simulink model "RRRplanaire"  (R2023a)
settings: Solver=ode23  StartTime=0.0  StopTime=10  FixedStep=.1  RelTol=1e-3  EnableMultiTasking=on
values from neighbouring files (symbols this model uses):
  A = 0.1    [Boucle.m]    (also in param.m)
  w = 1    [Boucle.m]    (also in param.m)
  x0 = 0.4    [Boucle.m]    (also in param.m)
  y0 = 0.3    [Boucle.m]    (also in param.m)
libraries: vrlib x4, dspsolvers x1
settings Model: Creator=dgarcia  LastModifiedBy=maxim
settings SolverCC: AlgebraicLoopSolver=TrustRegion
settings DataIOCC: LimitDataPoints=on  SaveFormat=Array  SignalLoggingSaveFormat=ModelDataLogs  ReturnWorkspaceOutputs=off  SignalLoggingName=sigsOut
settings OptimizationCC: ExpressionDepthLimit=2147483647  InitFltsAndDblsToZero=on  LifeSpan=inf
settings DebuggingCC: SaveWithParameterizedLinksMsg=none  UnderspecifiedInitializationDetection=Classic  MergeDetectMultiDrivingBlocksExec=none  SignalResolutionControl=TryResolveAllWithWarning  MultiTaskDSMMsg=warning  MultiTaskCondExecSysMsg=none  FcnCallInpInsideContextMsg=warning  UnconnectedInputMsg=warning  UnconnectedOutputMsg=warning  UnconnectedLineMsg=warning  StateNameClashWarn=warning  SFUnexpectedBacktrackingDiag=warning  SFNoUnconditionalDefaultTransitionDiag=warning  ArithmeticOperatorsInVariantConditions=warning
settings HardwareCC: ProdBitPerPointer=32  ProdBitPerSizeT=32  ProdBitPerPtrDiffT=32  ProdLargestAtomicFloat=None  ProdIntDivRoundTo=Undefined  ProdEndianess=Unspecified  ProdWordSize=32  ProdHWDeviceType=32-bit Generic  TargetUnknown=on
settings ModelReferenceCC: EnableRefExpFcnMdlSchedulingChecks=on  PropagateSignalLabelsOutOfModel=off
settings SFSimCC: SimUseLocalCustomCode=off  SimParseCustomCode=off  CustomCodeUndefinedFunction=UseInterfaceOnly
settings RTWCC: RTWUseLocalCustomCode=off  DLArmComputeVersion=19.05
settings CodeAppCC: StateflowObjectComments=on
settings GRTTargetCC: TargetFcnLib=ansi_tfl_tmw.mat  TargetLangStandard=C89/C90 (ANSI)  CombineOutputUpdateFcns=off  GRTInterface=on
settings ConfigComp: CovMetricSettings=dw  CovSaveCumulativeToWorkspaceVar=on  CovSaveSingleToWorkspaceVar=on  CovExternalEMLEnable=off

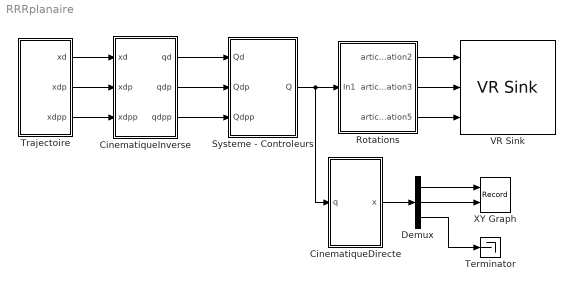
== system RRRplanaire ==
  CinematiqueDirecte : Subsystem
  CinematiqueInverse : Subsystem
  Demux : Demux  Outputs=3
  Rotations : Subsystem
  Systeme - Controleurs : Subsystem
  Terminator : Terminator
  Trajectoire : Subsystem
  VR Sink : vrlib/VR Sink  InstantiateOnLoad=on  SampleTime=0.1  ViewEnable=on  RemoteChange=off  RemoteView=on  FieldsWritten=Joint2.rotation.4.1.double#Joint3.rotation.4.1.double#Joint5.rotation.4.1.double  WorldFileName=LRMate200iC.wrl  AutoView=off  VideoDimensions=[]  AllowVariableSize=off
  XY Graph : Record  FileSettingsInternal="{\"entries\":[{\"content\":{\"excelSettings\":{\"content\":{},\"type\":\"Streamout.ExcelSettings\"}},\"type\":\"Streamout.FileSettingStorage\",\"uuid\":\"15e78eb5-29a8-49a9-9840-80e2d80b59b9\"}],\"packageUris\":[\"http://schema.mathworks.com/mf0/streamout_blocks/R2020a\"],\"version\":\"1.0\"}"  Layout=[1 1]  SignalsInternal="{\"entries\":[{\"content\":{\"signals\":[{\"content\":{\"blockPath\":[\"RRRplanaire/XY Graph\"],\"dimensions\":[1],\"domain\":\"RRRplanaire/XY Graph\",\"lineColor\":\"#a2142f\",\"plots\":[1],\"port\":1,\"signalID\":16,\"signalName\":\"XY Graph:1\"},\"type\":\"RecordBlkView.Signal\",\"uuid\":\"495b3c76-def4-49bc-ad31-84cb6030c742\"},{\"content\":{\"blockPath\":[\"RRRplanaire/XY Graph\"],\"dimensions\":[1],\"domain\":\"RRRplanaire/XY Graph\",\"lineColor\":\"#139fff\",\"plots\":[1],\"port\":2,\"signalID\":19,\"signalName\":\"XY Graph:2\"},\"type\":\"RecordBlkView.Signal\",\"uuid\":\"4d725a8f-b7c2-4f23-bdfe-d8f8ae9227f4\"}]},\"type\":\"RecordBlkView.InputSignals\",\"uuid\":\"0fe62230-b389-4f09-ad52-d3f22d0d1e4d\"}],\"packageUris\":[\"http://schema.mathworks.com/mf0/streamout_blocks/R2020a\"],\"version\":\"1.0\"}"  VisualizationBindings="{\"xyplotplugin\":{\"info\":[{\"series\":[{\"bindingParametersList\":[{\"parameter\":\"X-Axis\",\"signalID\":16,\"signalName\":\"XY Graph:1\"},{\"parameter\":\"Y-Axis\",\"signalID\":19,\"signalName\":\"XY Graph:2\"}],\"seriesID\":11629}],\"subplotID\":1}]}}"  CompatibilityTag=XY  st=-1
  wires:
  Systeme - Controleurs/1(Q) -> CinematiqueDirecte/1(q), Rotations/1(In1)
  Trajectoire/1(xd) -> CinematiqueInverse/1(xd)
  Trajectoire/3(xdpp) -> CinematiqueInverse/3(xdpp)
  CinematiqueInverse/3(qdpp) -> Systeme - Controleurs/3(Qdpp)
  Trajectoire/2(xdp) -> CinematiqueInverse/2(xdp)
  CinematiqueInverse/1(qd) -> Systeme - Controleurs/1(Qd)
  CinematiqueInverse/2(qdp) -> Systeme - Controleurs/2(Qdp)
  CinematiqueDirecte/1(x) -> Demux/1
  Demux/1 -> XY Graph/1
  Demux/2 -> XY Graph/2
  Demux/3 -> Terminator/1
  Rotations/1(articulation2) -> VR Sink/1
  Rotations/2(articulation3) -> VR Sink/2
  Rotations/3(articulation5) -> VR Sink/3

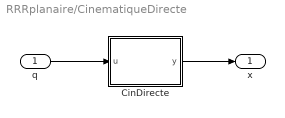
== system RRRplanaire/CinematiqueDirecte ==
  q : Inport
  CinDirecte : MATLAB Function  TreatAsAtomicUnit=on
  x : Outport
  wires:
  q/1 -> CinDirecte/1(u)
  CinDirecte/1(y) -> x/1

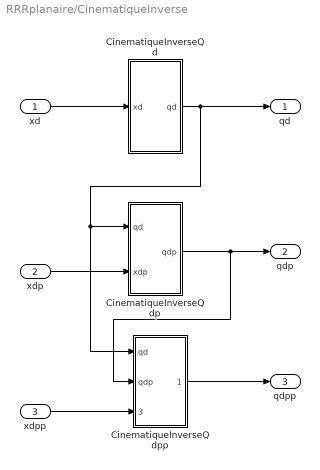
== system RRRplanaire/CinematiqueInverse ==
  xd : Inport
  xdp : Inport  Port=2
  xdpp : Inport  Port=3
  CinematiqueInverseQd : Subsystem
  CinematiqueInverseQdp : Subsystem
  CinematiqueInverseQdpp : Subsystem
  qd : Outport
  qdp : Outport  Port=2
  qdpp : Outport  Port=3
  wires:
  CinematiqueInverseQd/1(qd) -> CinematiqueInverseQdp/1(qd), CinematiqueInverseQdpp/1(qd), qd/1
  xdp/1 -> CinematiqueInverseQdp/2(xdp)
  CinematiqueInverseQdp/1(qdp) -> qdp/1, CinematiqueInverseQdpp/2(qdp)
  xd/1 -> CinematiqueInverseQd/1(xd)
  CinematiqueInverseQdpp/1(qdpp) -> qdpp/1
  xdpp/1 -> CinematiqueInverseQdpp/3(xdpp)

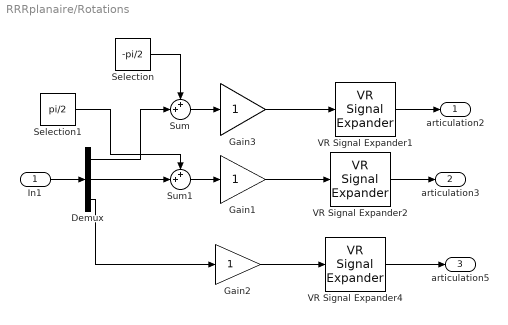
== system RRRplanaire/Rotations ==
  In1 : Inport
  Demux : Demux  Outputs=3
      settings: DisplayOption=none
  Gain1 : Gain
  Gain2 : Gain
  Gain3 : Gain
  Selection : Constant  Value=-pi/2  VectorParams1D=off
  Selection1 : Constant  Value=pi/2  VectorParams1D=off
  Sum : Sum  Inputs=++|
  Sum1 : Sum  Inputs=++|
  VR Signal Expander1 : vrlib/VR Signal Expander  outwidth=4  outidx=4
  VR Signal Expander2 : vrlib/VR Signal Expander  outwidth=4  outidx=4
  VR Signal Expander4 : vrlib/VR Signal Expander  outwidth=4  outidx=4
  articulation2 : Outport
  articulation3 : Outport  Port=2
  articulation5 : Outport  Port=3
  wires:
  In1/1 -> Demux/1
  VR Signal Expander1/1 -> articulation2/1
  VR Signal Expander2/1 -> articulation3/1
  Gain1/1 -> VR Signal Expander2/1
  Gain3/1 -> VR Signal Expander1/1
  VR Signal Expander4/1 -> articulation5/1
  Demux/3 -> Gain2/1
  Gain2/1 -> VR Signal Expander4/1
  Selection/1 -> Sum/1
  Demux/1 -> Sum/2
  Sum/1 -> Gain3/1
  Demux/2 -> Sum1/2
  Sum1/1 -> Gain1/1
  Selection1/1 -> Sum1/1

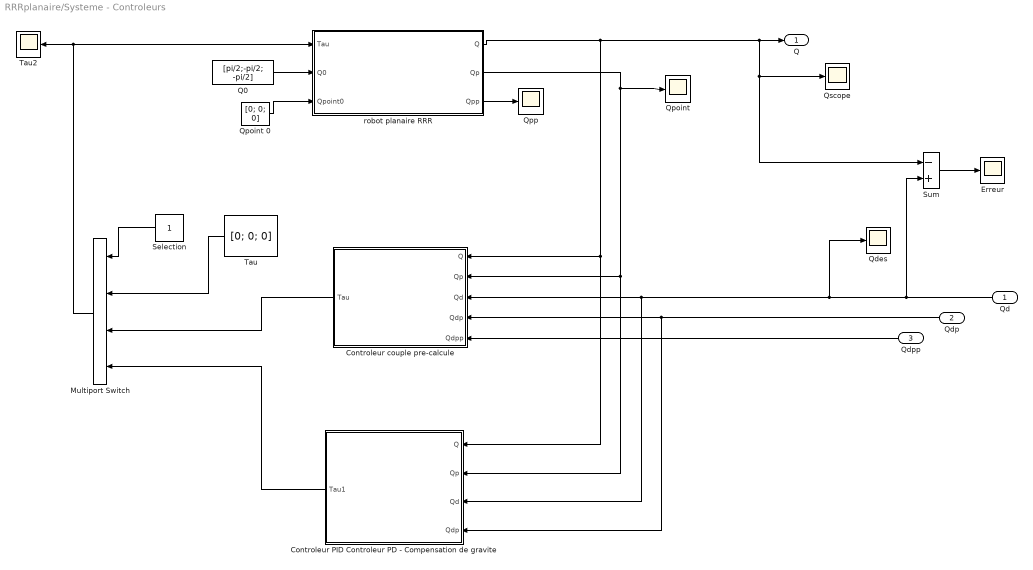
== system RRRplanaire/Systeme - Controleurs ==
  Qd : Inport
  Qdp : Inport  Port=2
  Qdpp : Inport  Port=3
  Controleur PID Controleur PD - Compensation de gravite : Subsystem
  Controleur couple pre-calcule : Subsystem
  Erreur : Scope
  Multiport Switch : MultiPortSwitch  InputSameDT=off
  "Q0 " : Constant  Value=[pi/2;-pi/2; -pi/2]  VectorParams1D=off
  Qdes : Scope
  Qpoint : Scope
  "Qpoint 0  " : Constant  Value=[0; 0; 0]  VectorParams1D=off
  Qpp : Scope
  Qscope : Scope
  Selection : Constant  VectorParams1D=off
  Sum : Sum  Inputs=-+  SaturateOnIntegerOverflow=on
  Tau : Constant  Value=[0; 0; 0]  VectorParams1D=off
  Tau2 : Scope
  robot planaire RRR : Subsystem
  Q : Outport
  wires:
  "Q0 "/1 -> robot planaire RRR/2(Q0)
  "Qpoint 0  "/1 -> robot planaire RRR/3(Qpoint0)
  robot planaire RRR/1(Q) -> Sum/1, Qscope/1, Q/1, Controleur couple pre-calcule/1(Q), Controleur PID Controleur PD - Compensation de gravite/1(Q)
  robot planaire RRR/2(Qp) -> Qpoint/1, Controleur PID Controleur PD - Compensation de gravite/2(Qp), Controleur couple pre-calcule/2(Qp)
  Sum/1 -> Erreur/1
  Controleur couple pre-calcule/1(Tau) -> Multiport Switch/3
  Tau/1 -> Multiport Switch/2
  Selection/1 -> Multiport Switch/1
  Controleur PID Controleur PD - Compensation de gravite/1(Tau1) -> Multiport Switch/4
  Qd/1 -> Sum/2, Controleur couple pre-calcule/3(Qd), Controleur PID Controleur PD - Compensation de gravite/3(Qd), Qdes/1
  Multiport Switch/1 -> Tau2/1, robot planaire RRR/1(Tau)
  Qdp/1 -> Controleur couple pre-calcule/4(Qdp), Controleur PID Controleur PD - Compensation de gravite/4(Qdp)
  Qdpp/1 -> Controleur couple pre-calcule/5(Qdpp)
  robot planaire RRR/3(Qpp) -> Qpp/1

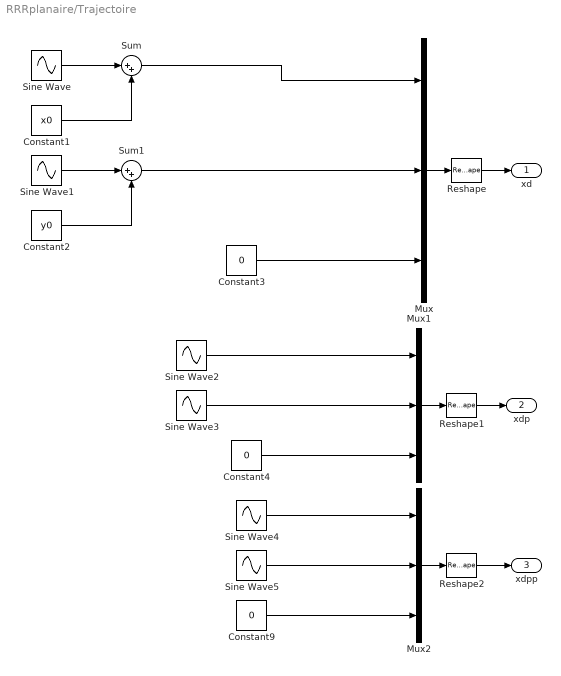
== system RRRplanaire/Trajectoire ==
  Constant1 : Constant  Value=x0
  Constant2 : Constant  Value=y0
  Constant3 : Constant  Value=0
  Constant4 : Constant  Value=0
  Constant9 : Constant  Value=0
  Mux : Mux  Inputs=3
  Mux1 : Mux  Inputs=3
  Mux2 : Mux  Inputs=3
  Reshape : Reshape  OutputDimensionality=Column vector (2-D)
  Reshape1 : Reshape  OutputDimensionality=Column vector (2-D)
  Reshape2 : Reshape  OutputDimensionality=Column vector (2-D)
  Sine Wave : Sin  Amplitude=A  Frequency=w  Phase=-pi/2  SampleTime=0
  Sine Wave1 : Sin  Amplitude=A  Frequency=w  SampleTime=0
  Sine Wave2 : Sin  Amplitude=-A*w  Frequency=w  SampleTime=0
  Sine Wave3 : Sin  Amplitude=A*w  Frequency=w  Phase=-pi/2  SampleTime=0
  Sine Wave4 : Sin  Amplitude=-A*w^2  Frequency=w  Phase=-pi/2  SampleTime=0
  Sine Wave5 : Sin  Amplitude=-A*w^2  Frequency=w  SampleTime=0
  Sum : Sum  Inputs=|++
  Sum1 : Sum  Inputs=|++
  xd : Outport
  xdp : Outport  Port=2
  xdpp : Outport  Port=3
  wires:
  Mux/1 -> Reshape/1
  Mux1/1 -> Reshape1/1
  Mux2/1 -> Reshape2/1
  Reshape/1 -> xd/1
  Reshape1/1 -> xdp/1
  Reshape2/1 -> xdpp/1
  Sum1/1 -> Mux/2
  Constant3/1 -> Mux/3
  Sine Wave2/1 -> Mux1/1
  Sine Wave3/1 -> Mux1/2
  Sine Wave4/1 -> Mux2/1
  Sine Wave5/1 -> Mux2/2
  Constant9/1 -> Mux2/3
  Constant1/1 -> Sum/2
  Sine Wave/1 -> Sum/1
  Sum/1 -> Mux/1
  Sine Wave1/1 -> Sum1/1
  Constant2/1 -> Sum1/2
  Constant4/1 -> Mux1/3

== system RRRplanaire/CinematiqueInverse/CinematiqueInverseQd ==
  xd : Inport
  q2 : MATLAB Function  TreatAsAtomicUnit=on
  qd : Outport
  wires:
  q2/1(y) -> qd/1
  xd/1 -> q2/1(u)

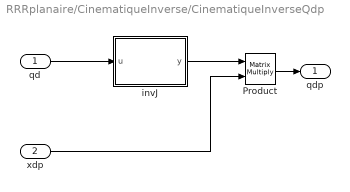
== system RRRplanaire/CinematiqueInverse/CinematiqueInverseQdp ==
  qd : Inport
  xdp : Inport  Port=2
  Product : Product  Multiplication=Matrix(*)  RndMeth=Zero
  invJ : MATLAB Function  TreatAsAtomicUnit=on
  qdp : Outport
  wires:
  xdp/1 -> Product/2
  qd/1 -> invJ/1(u)
  invJ/1(y) -> Product/1
  Product/1 -> qdp/1

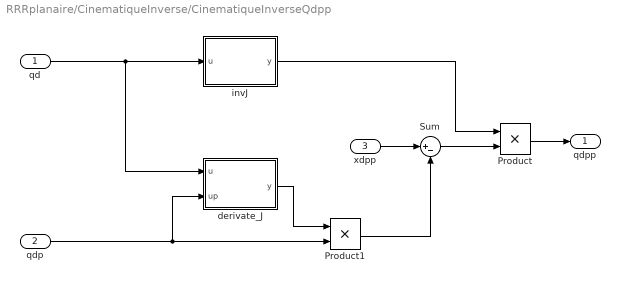
== system RRRplanaire/CinematiqueInverse/CinematiqueInverseQdpp ==
  qd : Inport
  qdp : Inport  Port=2
  xdpp : Inport  Port=3
  Product : Product
  Product1 : Product
  Sum : Sum  Inputs=|+-
  derivate_J : MATLAB Function  TreatAsAtomicUnit=on
  invJ : MATLAB Function  TreatAsAtomicUnit=on
  qdpp : Outport
  wires:
  qd/1 -> invJ/1(u), derivate_J/1(u)
  qdp/1 -> Product1/2, derivate_J/2(up)
  Product/1 -> qdpp/1
  xdpp/1 -> Sum/1
  derivate_J/1(y) -> Product1/1
  Product1/1 -> Sum/2
  Sum/1 -> Product/2
  invJ/1(y) -> Product/1

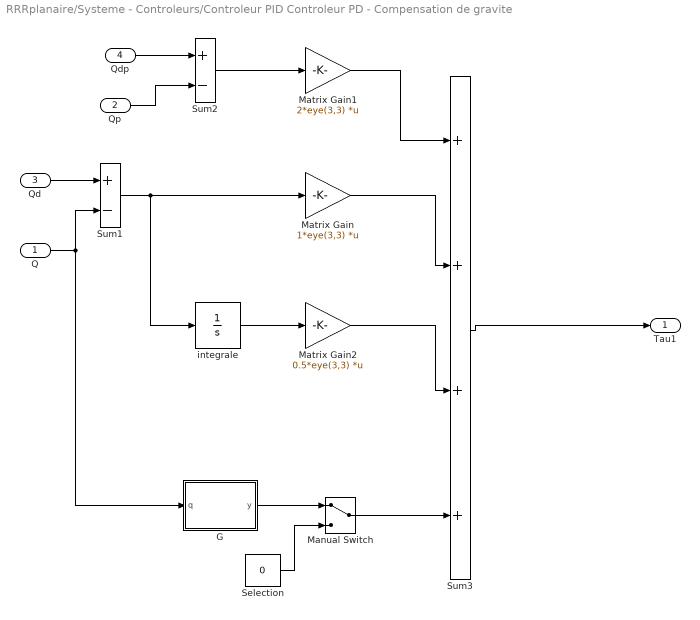
== system RRRplanaire/Systeme - Controleurs/Controleur PID Controleur PD - Compensation de gravite ==
  Q : Inport
  Qp : Inport  Port=2
  Qd : Inport  Port=3
  Qdp : Inport  Port=4
  G : MATLAB Function  TreatAsAtomicUnit=on
  Manual Switch : ManualSwitch
  Matrix Gain : Gain  Gain=1*eye(3,3)  Multiplication=Matrix(K*u)  SaturateOnIntegerOverflow=on  OutDataTypeStr=Inherit: Same as input  ParamDataTypeStr=Inherit: Same as input
  Matrix Gain1 : Gain  Gain=2*eye(3,3)  Multiplication=Matrix(K*u)  SaturateOnIntegerOverflow=on  OutDataTypeStr=Inherit: Same as input  ParamDataTypeStr=Inherit: Same as input
  Matrix Gain2 : Gain  Gain=0.5*eye(3,3)  Multiplication=Matrix(K*u)  SaturateOnIntegerOverflow=on  OutDataTypeStr=Inherit: Same as input  ParamDataTypeStr=Inherit: Same as input
  Selection : Constant  Value=0  VectorParams1D=off
  Sum1 : Sum  Inputs=+-  InputSameDT=on  SaturateOnIntegerOverflow=on  OutDataTypeStr=Inherit: Same as first input
  Sum2 : Sum  Inputs=+-  InputSameDT=on  SaturateOnIntegerOverflow=on  OutDataTypeStr=Inherit: Same as first input
  Sum3 : Sum  Inputs=++++  InputSameDT=on  SaturateOnIntegerOverflow=on  OutDataTypeStr=Inherit: Same as first input
  integrale : Integrator  InitialCondition=[0; 0; 0]
  Tau1 : Outport
  wires:
  Selection/1 -> Manual Switch/2
  G/1(y) -> Manual Switch/1
  Manual Switch/1 -> Sum3/4
  Sum3/1 -> Tau1/1
  Matrix Gain2/1 -> Sum3/3
  Matrix Gain/1 -> Sum3/2
  Matrix Gain1/1 -> Sum3/1
  integrale/1 -> Matrix Gain2/1
  Qdp/1 -> Sum2/1
  Sum2/1 -> Matrix Gain1/1
  Sum1/1 -> integrale/1, Matrix Gain/1
  Qd/1 -> Sum1/1
  Qp/1 -> Sum2/2
  Q/1 -> G/1(q), Sum1/2

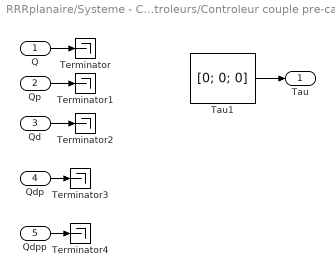
== system RRRplanaire/Systeme - Controleurs/Controleur couple pre-calcule ==
  Q : Inport
  Qp : Inport  Port=2
  Qd : Inport  Port=3
  Qdp : Inport  Port=4
  Qdpp : Inport  Port=5
  Tau1 : Constant  Value=[0; 0; 0]  VectorParams1D=off
  Terminator{,1..4} (5 alike) : Terminator
  Tau : Outport
  wires:
  Qdpp/1 -> Terminator4/1
  Qdp/1 -> Terminator3/1
  Q/1 -> Terminator/1
  Qp/1 -> Terminator1/1
  Qd/1 -> Terminator2/1
  Tau1/1 -> Tau/1

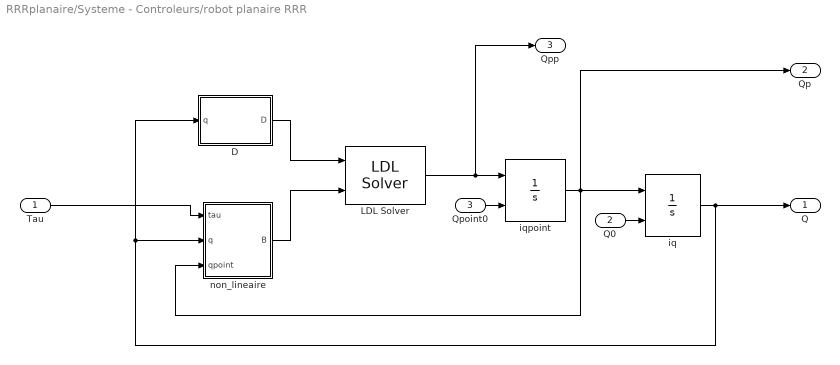
== system RRRplanaire/Systeme - Controleurs/robot planaire RRR ==
  Tau : Inport
  Q0 : Inport  Port=2
  Qpoint0 : Inport  Port=3
  "D " : MATLAB Function  TreatAsAtomicUnit=on
  LDL Solver : dspsolvers/LDL Solver  errmode=Warning
  iq : Integrator  InitialConditionSource=external  InitialCondition=[0;-pi/2; 0]
  iqpoint : Integrator  InitialConditionSource=external  InitialCondition=[0; 0; 0]
  non_lineaire : Subsystem
  Q : Outport
  Qp : Outport  Port=2
  Qpp : Outport  Port=3
  wires:
  "D "/1(D) -> LDL Solver/1
  non_lineaire/1(B) -> LDL Solver/2
  LDL Solver/1 -> iqpoint/1, Qpp/1
  iq/1 -> "D "/1(q), non_lineaire/2(q), Q/1
  Q0/1 -> iq/2
  iqpoint/1 -> iq/1, Qp/1, non_lineaire/3(qpoint)
  Qpoint0/1 -> iqpoint/2
  Tau/1 -> non_lineaire/1("tau ")

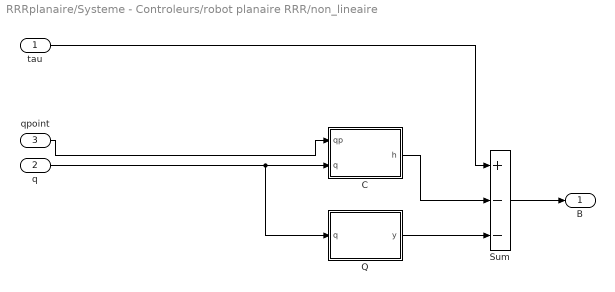
== system RRRplanaire/Systeme - Controleurs/robot planaire RRR/non_lineaire ==
  "tau " : Inport
  q : Inport  Port=2
  qpoint : Inport  Port=3
  C : MATLAB Function  TreatAsAtomicUnit=on
  "Q " : MATLAB Function  TreatAsAtomicUnit=on
  Sum : Sum  Inputs=+--  InputSameDT=on  SaturateOnIntegerOverflow=on  OutDataTypeStr=Inherit: Same as first input
  B : Outport
  wires:
  q/1 -> "Q "/1(q), C/2(q)
  "tau "/1 -> Sum/1
  Sum/1 -> B/1
  "Q "/1(y) -> Sum/3
  C/1(h) -> Sum/2
  qpoint/1 -> C/1(qp)

== matlab function RRRplanaire/Systeme - Controleurs/Controleur PID Controleur PD - Compensation de gravite/G ==
  data: q input; y output
function y = fcn(q)

% Paramètres
M1 = 1;
M2 = 1;
M3 = 0.5;
L1 = 300*0.001;
L2 = 320*0.001;
L3 = 80*0.001;
g = 9.81;
T = 0.01;


I1 = 1/12*M1*L1^2;
I2 = 1/12*M2*L2^2;
I3 = 1/12*M3*L3^2;
C1 = L1/2;
C2 = L2/2;
C3 = L3/2;
p1 = M1*C1^2+I1+(M2+M3)*L1^2;
p2 = M2*C2^2+I2+M3*L2^2;
p3 = M3*C3^2+I3;
p4 = (M2+2*M3)*L1*L2/2;
p5 = M3*L1*L3/2;
p6 = M3*L2*L3/2;
p7 = (M1*C1+(M2+M3)*L1)*g;
p8 = (M2*C2+M3*L2)*g;
p9 = M3*C3*g;

y = [p7*cos(q(1))+p8*cos(q(1)+q(2))+p9*cos(q(1)+q(2)+q(3))
     p8*cos(q(1)+q(2))+p9*cos(q(1)+q(2)+q(3))
     p9*cos(q(1)+q(2)+q(3))];

== matlab function RRRplanaire/CinematiqueInverse/CinematiqueInverseQdpp/derivate_J ==
  data: u input; y output; up input
function y = fcn(u,up)

% Paramètres
L1 = 300*0.001;
L2 = 320*0.001;
L3 = 80*0.001;

y=[-L3 * cos(u(1) + u(2) + u(3))*(up(1)+up(2)+up(3)) - L2 * cos(u(1) + u(2))*(up(1)+up(2)) - L1 * cos(u(1))*up(1), -L3 * cos(u(1) + u(2) + u(3))*(up(1)+up(2)+up(3)) - L2 * cos(u(1) + u(2))*(up(1)+up(2)), -L3 * cos(u(1) + u(2) + u(3))*(up(1)+up(2)+up(3)); 
   -L3 * sin(u(1) + u(2) + u(3))*(up(1)+up(2)+up(3)) - L2 * sin(u(1) + u(2))*(up(1)+up(2)) - L1 * sin(u(1))*up(1), -L3 * sin(u(1) + u(2) + u(3))*(up(1)+up(2)+up(3)) - L2 * sin(u(1) + u(2))*(up(1)+up(2)), -L3 * sin(u(1) + u(2) + u(3))*(up(1)+up(2)+up(3));
   1 1 1;];

== matlab function RRRplanaire/Systeme - Controleurs/robot planaire RRR/D  ==
  data: q input; D output
function D = fcn(q)

% Paramètres
M1 = 1;
M2 = 1;
M3 = 0.5;
L1 = 300*0.001;
L2 = 320*0.001;
L3 = 80*0.001;
g = 9.81;
T = 0.01;

I1 = 1/12*M1*L1^2;
I2 = 1/12*M2*L2^2;
I3 = 1/12*M3*L3^2;
C1 = L1/2;
C2 = L2/2;
C3 = L3/2;
p1 = M1*C1^2+I1+(M2+M3)*L1^2;
p2 = M2*C2^2+I2+M3*L2^2;
p3 = M3*C3^2+I3;
p4 = (M2+2*M3)*L1*L2/2;
p5 = M3*L1*L3/2;
p6 = M3*L2*L3/2;
p7 = (M1*C1+(M2+M3)*L1)*g;
p8 = (M2*C2+M3*L2)*g;
p9 = M3*C3*g;

D = [p1+p2+p3+2*p4*cos(q(2))+2*p5*cos(q(2)+q(3))+2*p6*cos(q(3)) p2+p3+p4*cos(q(2))+p5*cos(q(2)+q(3))+2*p6*cos(q(3)) p3+p5*cos(q(2)+q(3))+p6*cos(q(3))
     p2+p3+p4*cos(q(2))+p5*cos(q(2)+q(3))+2*p6*cos(q(3)) p2+p3+2*p6*cos(q(3)) p3+p6*cos(q(3))
     p3+p5*cos(q(2)+q(3))+p6*cos(q(3)) p3+p6*cos(q(3)) p3];

== matlab function RRRplanaire/Systeme - Controleurs/robot planaire RRR/non_lineaire/C ==
  data: qp input; h output; q input
function h = fcn(qp,q)

% Paramètres
M1 = 1;
M2 = 1;
M3 = 0.5;
L1 = 300*0.001;
L2 = 320*0.001;
L3 = 80*0.001;
g = 9.81;
T = 0.01;

I1 = 1/12*M1*L1^2;
I2 = 1/12*M2*L2^2;
I3 = 1/12*M3*L3^2;
C1 = L1/2;
C2 = L2/2;
C3 = L3/2;
p1 = M1*C1^2+I1+(M2+M3)*L1^2;
p2 = M2*C2^2+I2+M3*L2^2;
p3 = M3*C3^2+I3;
p4 = (M2+2*M3)*L1*L2/2;
p5 = M3*L1*L3/2;
p6 = M3*L2*L3/2;
p7 = (M1*C1+(M2+M3)*L1)*g;
p8 = (M2*C2+M3*L2)*g;
p9 = M3*C3*g;

h = [-p4*(2*qp(1)+qp(2))*qp(2)*sin(q(2))-p5*(qp(2)+qp(3))*(2*qp(1)+qp(2)+qp(3))*sin(q(2)+q(3))-p6*qp(3)*(2*qp(1)+2*qp(2)+qp(3))*sin(q(3))
     p4*sin(q(2))*qp(1)^2+p5*sin(q(2)+q(3))*qp(1)^2-p6*(2*qp(1)+2*qp(2)+qp(3))*qp(3)*sin(q(3))
     p5*sin(q(2)+q(3))*qp(1)^2+p6*sin(q(3))*(qp(1)+qp(2))^2];

== matlab function RRRplanaire/Systeme - Controleurs/robot planaire RRR/non_lineaire/Q  ==
  data: q input; y output
function y = fcn(q)

% Paramètres
M1 = 1;
M2 = 1;
M3 = 0.5;
L1 = 300*0.001;
L2 = 320*0.001;
L3 = 80*0.001;
g = 9.81;
T = 0.01;

I1 = 1/12*M1*L1^2;
I2 = 1/12*M2*L2^2;
I3 = 1/12*M3*L3^2;
C1 = L1/2;
C2 = L2/2;
C3 = L3/2;
p1 = M1*C1^2+I1+(M2+M3)*L1^2;
p2 = M2*C2^2+I2+M3*L2^2;
p3 = M3*C3^2+I3;
p4 = (M2+2*M3)*L1*L2/2;
p5 = M3*L1*L3/2;
p6 = M3*L2*L3/2;
p7 = (M1*C1+(M2+M3)*L1)*g;
p8 = (M2*C2+M3*L2)*g;
p9 = M3*C3*g;

y = [p7*cos(q(1))+p8*cos(q(1)+q(2))+p9*cos(q(1)+q(2)+q(3))
     p8*cos(q(1)+q(2))+p9*cos(q(1)+q(2)+q(3))
     p9*cos(q(1)+q(2)+q(3))];

== matlab function RRRplanaire/CinematiqueInverse/CinematiqueInverseQd/q2 ==
  data: u input; y output
function y = fcn(u)
% u(1) = Ex_d, u(2) = Ey_d, u(3) = theta_d
% y(1) = theta(1), y(2) = theta(2), y(3) = theta(3)

% Paramètres
l1 = 300*0.001;
l2 = 320*0.001;
l3 = 80*0.001;

xd = u(1);
yd = u(2);
phi_des = u(3);
Wx = xd - l3*cos(phi_des);
Wy = yd - l3*sin(phi_des);
d = sqrt(Wx^2+Wy^2);
theta1 = atan2(Wy,Wx) + acos((d^2+l1^2-l2^2)/(2*d*l1));
theta2 = -acos((d^2-l1^2-l2^2)/(2*l1*l2));
theta3 = phi_des - theta2- theta1;

y=[theta1, theta2, theta3];

== matlab function RRRplanaire/CinematiqueInverse/CinematiqueInverseQdp/invJ ==
  data: u input; y output
function y = fcn(u)

% Paramètres
L1 = 300*0.001;
L2 = 320*0.001;
L3 = 80*0.001;

J=[-L3 * sin(u(1) + u(2) + u(3)) - L2 * sin(u(1) + u(2)) - L1 * sin(u(1)) -L3 * sin(u(1) + u(2) + u(3)) - L2 * sin(u(1) + u(2)) -L3 * sin(u(1) + u(2) + u(3)); L3 * cos(u(1) + u(2) + u(3)) + L2 * cos(u(1) + u(2)) + L1 * cos(u(1)) L3 * cos(u(1) + u(2) + u(3)) + L2 * cos(u(1) + u(2)) L3 * cos(u(1) + u(2) + u(3)); 1 1 1;];
y=inv(J);

== matlab function RRRplanaire/CinematiqueDirecte/CinDirecte ==
  data: u input; y output
function y = fcn(u)
% y(1) = Ex, y(2) = Ey, y(3) = theta
% u(1) = theta(1), u(2) = theta(2), u(3) = theta(3)

% Lea parametres du robot, M1, M2, M3, L1, L2, L3, g et T
% sont définis dans les fichiers de la dynamique par exemple
% Ces paramètres peuvent être copiés-collés ici
l1 = 300*0.001;
l2 = 320*0.001;
l3 = 80*0.001;
t1 = u(1);
t2 = u(2);
t3= u(3);

y = [cos(t1+t2+t3) -sin(t1+t2+t3) l3*cos(t1+t2+t3)+l2*cos(t1+t2)+l1*cos(t1);
        sin(t1+t2+t3) cos(t1+t2+t3) l3*sin(t1+t2+t3)+l2*sin(t1+t2)+l1*sin(t1);
        0 0 1];

== matlab function RRRplanaire/CinematiqueInverse/CinematiqueInverseQdpp/invJ ==
  data: u input; y output
function y = fcn(u)

% Paramètres
L1 = 300*0.001;
L2 = 320*0.001;
L3 = 80*0.001;

J=[-L3 * sin(u(1) + u(2) + u(3)) - L2 * sin(u(1) + u(2)) - L1 * sin(u(1)) -L3 * sin(u(1) + u(2) + u(3)) - L2 * sin(u(1) + u(2)) -L3 * sin(u(1) + u(2) + u(3)); L3 * cos(u(1) + u(2) + u(3)) + L2 * cos(u(1) + u(2)) + L1 * cos(u(1)) L3 * cos(u(1) + u(2) + u(3)) + L2 * cos(u(1) + u(2)) L3 * cos(u(1) + u(2) + u(3)); 1 1 1;];
y=;
